simulink model "Jakub_Adamczyk_model1"  (Simulink 8.0)
settings: Solver=ode45  StartTime=0.0  StopTime=20  RelTol=1e-3
values from neighbouring files (symbols this model uses):
  Amplituda = 1    [Jakub_Adamczyk_skrypt.m]
  Czestotliwosc = 5    [Jakub_Adamczyk_skrypt.m]
settings Model: Creator=Jakub Adamczyk  LastModifiedBy=Jakub Adamczyk
settings DataIOCC: LimitDataPoints=off

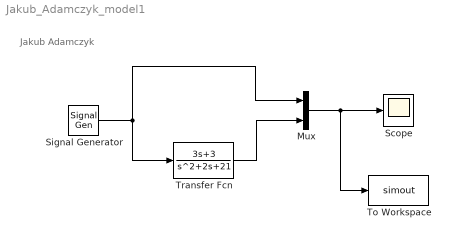
== system Jakub_Adamczyk_model1 ==
  note: Jakub Adamczyk
  Mux : Mux  Inputs=2
  Scope : Scope
  Signal Generator : SignalGenerator  Amplitude=Amplituda  Frequency=Czestotliwosc
  To Workspace : ToWorkspace  VariableName=simout  SampleTime=-1
  Transfer Fcn : TransferFcn  Numerator=[3 3]  Denominator=[1 2 21]
  wires:
  Signal Generator/1 -> Mux/1, Transfer Fcn/1
  Transfer Fcn/1 -> Mux/2
  Mux/1 -> To Workspace/1, Scope/1
